simulink model "ARB_ACTIVE_LQR."  (R2020a)
settings: Solver=FixedStepAuto  StartTime=0.0  StopTime=10  FixedStep=0.01  RelTol=1e-3
undefined symbols (not defined in the file or in its folder): A_ativo, B_ativo, D_ativo, K_r, sigbuilder_block, T
settings Model: Creator=Vitor  LastModifiedBy=Vitor
settings DebuggingCC: UnconnectedInputMsg=none  UnconnectedOutputMsg=none  UnconnectedLineMsg=none
settings ModelReferenceCC: EnableRefExpFcnMdlSchedulingChecks=off
settings RTWCC: Description=Generic Real-Time Target

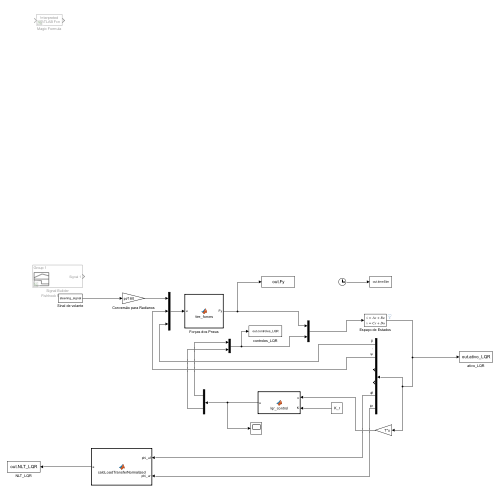
[thumbnail: Simulink's stored preview of the top-level diagram]
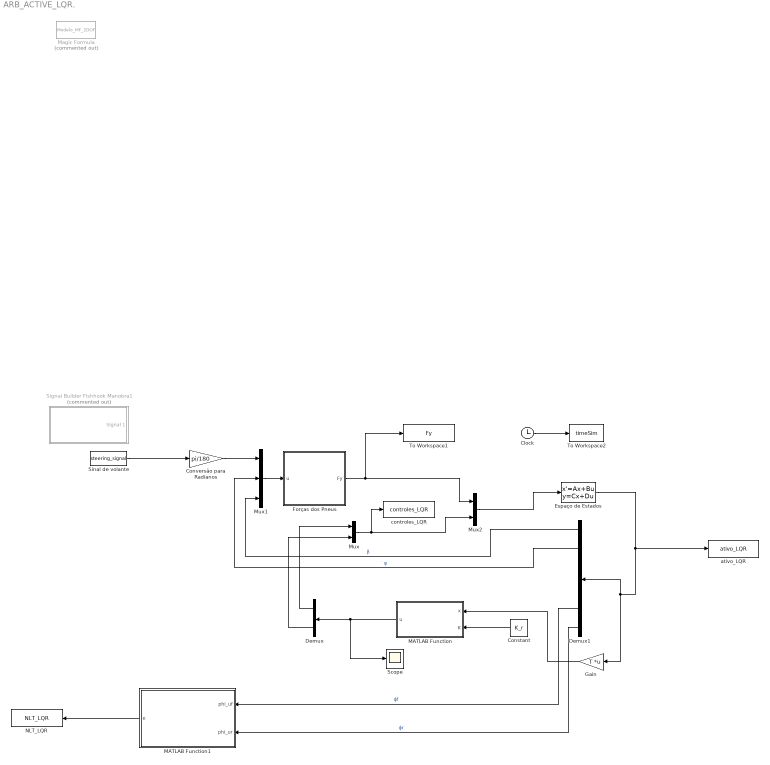
== system ARB_ACTIVE_LQR. ==
  Clock : Clock
  Constant : Constant  Value=K_r
  Conversão para Radianos : Gain  Gain=pi/180
  Demux : Demux  Outputs=2
  Demux1 : Demux  Outputs=6
  Espaço de Estados : StateSpace  A=A_ativo  B=B_ativo  C=eye(6)  D=D_ativo  InitialCondition=0
  Forças dos Pneus : MATLAB Function  TreatAsAtomicUnit=on
  Gain : Gain  Gain=T  Multiplication=Matrix(K*u)
  MATLAB Function : MATLAB Function  TreatAsAtomicUnit=on
  MATLAB Function1 : MATLAB Function  TreatAsAtomicUnit=on
  Magic Formula : MATLABFcn  Commented=on  MATLABFcn=Modelo_MF_2DOF  OutputDimensions=2
  Mux : Mux  Inputs=2
  Mux1 : Mux  Inputs=3
  Mux2 : Mux  Inputs=2
  NLT_LQR : ToWorkspace  VariableName=NLT_LQR  SampleTime=-1
  Scope : Scope
  Signal Builder Fishhook Manobra1 : Subsystem  Tag=STV Subsys  Commented=on  LoadFcn=sigbuilder_block('load');  StartFcn=sigbuilder_block('start');  StopFcn=sigbuilder_block('stop');  ClipboardFcn=sigbuilder_block('clipboard');  mask(Sigbuilder block){tuvar=[0:10]}
      mask help: Simulink:masks:SigbuilderBlock_MD
      mask init:
      | if ~strcmp(get_param(bdroot(gcbh),'SimulationStatus'),'stopped') tuvar = sigbuilder_block('maskInit'); end
      settings: CopyFcn=sigbuilder_block('copy');  DeleteFcn=sigbuilder_block('delete');  ModelCloseFcn=sigbuilder_block('modelClose');  PreSaveFcn=sigbuilder_block('preSave');  PauseFcn=sigbuilder_block('pause');  ContinueFcn=sigbuilder_block('continue');  NameChangeFcn=sigbuilder_block('namechange');  OpenFcn=sigbuilder_block('open',[17.4 79.8 1141.2 438.6 ]);  CloseFcn=sigbuilder_block('close');
      mask Display: plot(0, 0, 100, 100,[2, 2, 32, 32, 2], [68, 8, 8, 68, 68],[32, 2], [38, 38], [32, 19, 2],[53, 60, 44], [32, 17, 17, 2],[16, 16, 31, 31]);txt = getActiveGroup(gcbh);text(2, 100, txt,'verticalAlignment', 'top');
  Sinal de volante : FromWorkspace  VariableName=steering_signal
  To Workspace1 : ToWorkspace  VariableName=Fy  SampleTime=-1
  To Workspace2 : ToWorkspace  VariableName=timeSim  SampleTime=-1
  ativo_LQR : ToWorkspace  VariableName=ativo_LQR  SampleTime=-1
  controles_LQR : ToWorkspace  VariableName=controles_LQR  SampleTime=-1
  wires:
  Sinal de volante/1 -> Conversão para Radianos/1
  Clock/1 -> To Workspace2/1
  Conversão para Radianos/1 -> Mux1/1
  Mux1/1 -> Forças dos Pneus/1(u)
  Demux1/2 -> Mux1/2  "˙ ψ"
  Demux1/1 -> Mux1/3  "β"
  Forças dos Pneus/1(Fy) -> To Workspace1/1, Mux2/1
  Mux2/1 -> Espaço de Estados/1
  Espaço de Estados/1 -> Gain/1, Demux1/1, ativo_LQR/1
  Mux/1 -> Mux2/2, controles_LQR/1
  MATLAB Function/1(u) -> Scope/1, Demux/1
  Constant/1 -> MATLAB Function/2(K)
  Demux/1 -> Mux/1
  Demux/2 -> Mux/2
  Gain/1 -> MATLAB Function/1(x)
  Demux1/5 -> MATLAB Function1/1(phi_uf)  "ϕf"
  Demux1/6 -> MATLAB Function1/2(phi_ur)  "ϕr"
  MATLAB Function1/1(e) -> NLT_LQR/1

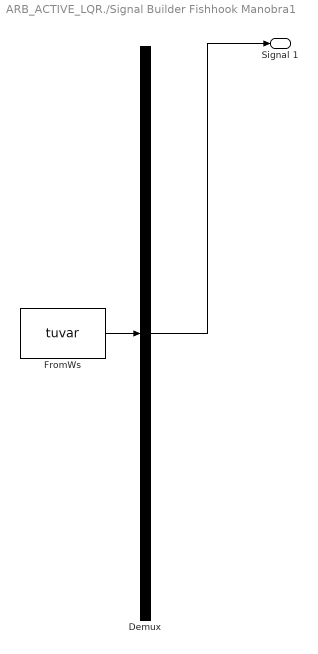
== system ARB_ACTIVE_LQR./Signal Builder Fishhook Manobra1 ==
  Demux : Demux  Tag=STV Demux  Outputs=1
      settings: DisplayOption=none
  FromWs : FromWorkspace  Tag=STV FromWs  VariableName=tuvar
      SigBuilderData=|
      | common.afterFinalStr = 'Extrapolate'
      | common.sampleTime = 0
      | dataSet.timeRange = [0 10]
      | dataSet.name = 'Group 1'
      | sbobj.Groups.Name = 'Group 1'
      | sbobj.Groups.Signals.Name = 'Signal 1'
      | sbobj.Groups.Signals.XData = [0 1 1.25 1.5 2 5 9 10]
      | sbobj.Groups.Signals.YData = [0 0 10 10 -10 -10 0 0]
  Signal 1 : Outport  Tag=STV Outport
  wires:
  Demux/1 -> Signal 1/1
  FromWs/1 -> Demux/1

== matlab function ARB_ACTIVE_LQR./Forças dos Pneus ==
  data: Fy output; u input
% Function: tire_forces.m
% Description: Calculate tire lateral forces using slip angles

function Fy  = tire_forces(u)
    % Descrição das Entradas
    beta = u(3);        % Ângulo de Deriva
    psi_dot = u(2);     % Taxa de Guinada
    delta_f = u(1);     % Ângulo de Esterçamento
    
    % Parâmetros do veículo (fixos na função para evitar problemas de escopo)
    lf = 1.95;           % Distância do CG ao eixo dianteiro (m)
    lr = 1.54;           % Distância do CG ao eixo traseiro (m)
    Cf = 582000;         % Rigidez lateral do pneu dianteiro (N/rad)
    Cr = 783000;         % Rigidez lateral do pneu traseiro (N/rad)
    mu = 1;              % Coeficiente de aderência ao solo
    v = 70 / 3.6;        % Velocidade longitudinal (m/s)
    
    % Calcular ângulos de deriva
    alpha_f = -beta + delta_f - ((lf * psi_dot) / v);
    alpha_r = -beta + ((lr * psi_dot) / v);
    
    % Calcular forças laterais nos pneus (saídas escalares)
    Fyf = mu * Cf * alpha_f;
    Fyr = mu * Cr * alpha_r;

    % Combinar as saídas como vetor coluna (2x1)
    Fy = [Fyf; Fyr];
end

== matlab function ARB_ACTIVE_LQR./MATLAB Function1 ==
  data: phi_uf input; phi_ur input; e output
function e = calcLoadTransferNormalized(phi_uf, phi_ur)
% calcLoadTransferNormalized Calcula a transferência de carga normalizada
%   e = calcLoadTransferNormalized(phi_uf, phi_ur) retorna um vetor [ef, er]
%   onde ef e er são, respectivamente, a transferência de carga
%   normalizada nos eixos dianteiro e traseiro.
%
%   Entradas:
%     phi_uf – ângulo de roll da massa não suspensa dianteira (rad)
%     phi_ur – ângulo de roll da massa não suspensa traseira   (rad)
%
%   Saída:
%     e      – vetor 1×2: [e_front, e_rear]

    %% Parâmetros do veículo
    ms  = 1760;    % Massa suspensa (kg)
    muf = 61;      % Massa não suspensa dianteira (kg)
    mur = 53;      % Massa não suspensa traseira  (kg)
    m   = ms + muf + mur;      % Massa total (kg)
    g   = 9.81;               % Gravidade (m/s²)

    %% Geometria
    w   = 2.874;     % Wheelbase (m)
    lf  = 1.332;     % CG → eixo dianteiro (m)
    lr  = w - lf;    % CG → eixo traseiro  (m)
    lw  = w / 2;     % Metade da bitola (m)

    %% Rigidez de rolagem total (suspensão + anti-roll bar)
    Kf     = 95760.15;   % Suspensão dianteira (Nm/rad)
    kAO_f  = 10730;      % Barra dianteira     (Nm/rad)
    kf     = Kf + kAO_f; % Total dianteiro     (Nm/rad)

    Kr     = 53857.62;   % Suspensão traseira  (Nm/rad)
    kAO_r  = 15480;      % Barra traseira      (Nm/rad)
    kr     = Kr + kAO_r; % Total traseiro      (Nm/rad)

    %% Transferência normalizada – dianteiro
    deltaFzf       = (kf * phi_uf) / lw;          % variação de carga vertical (N)
    Fzf            = (m * g * lr) / (lf + lr);    % carga estática estática (N)
    e_front        = deltaFzf / Fzf;              % normalizada

    %% Transferência normalizada – traseiro
    deltaFzr       = (kr * phi_ur) / lw;          % variação de carga vertical (N)
    Fzr            = (m * g * lf) / (lf + lr);    % carga estática estática (N)
    e_rear         = deltaFzr / Fzr;              % normalizada

    %% Saída como vetor 1×2
    e = [e_front, e_rear];
end

== matlab function ARB_ACTIVE_LQR./MATLAB Function ==
  data: x input; u output; K input
function u = lqr_control(x, K)
% lqr_control - Calcula o sinal de controle baseado na lei de realimentação de estados LQR.
%
%   u = lqr_control(x) computa o sinal de controle u a partir do vetor de estados x,
%   usando a lei u = -K*x, onde K é a matriz de ganho obtida via LQR.
%
%   OBS.: A variável K deve estar disponível no workspace base, 
%         ou seja, você deverá ter calculado K anteriormente (por exemplo, via a função lqr).
%
%   Exemplo:
%       % Supondo que K já esteja definido no workspace
%       u = lqr_control(x);
%

% Calcula o sinal de controle
u = -K * x;
end
